simulink model "maglev"  (Simulink 3.00)
settings: Solver=ode45  StartTime=0.0  StopTime=10.0  RelTol=1e-3
values from neighbouring files (symbols this model uses):
  a = 0.2042    [mlevpar.m]
  b = 72.988    [mlevpar.m]
  g = 9.81    [mlevpar.m]
  mb = 0.0682    [mlevpar.m]
  yl = 0.02    [mlevpar.m]
settings Model: Creator=root

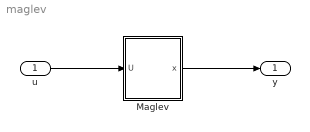
== system maglev ==
  u : Inport  Port=1  PortWidth=-1  SampleTime=-1  DataType=auto
      settings: SignalType=auto
  Maglev : Subsystem
  y : Outport  Port=1
  wires:
  Maglev/1(x) -> y/1
  u/1 -> Maglev/1(U)

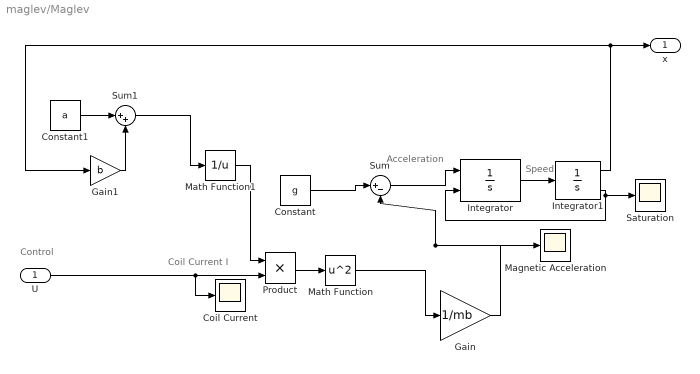
== system maglev/Maglev ==
  note: Control
  note: Speed
  note: Acceleration
  note: Coil Current I
  U : Inport  Port=1  PortWidth=-1  SampleTime=-1  DataType=auto
      settings: SignalType=auto
  Coil Current : Scope
      settings: TimeRange=auto  YMin=0  YMax=30  SaveToWorkspace=off  SaveName=ScopeData
  Constant : Constant  Value=g
  Constant1 : Constant  Value=a
  Gain : Gain  Gain=1/mb  SaturateOnIntegerOverflow=on
  Gain1 : Gain  Gain=b  SaturateOnIntegerOverflow=on
  Integrator : Integrator  ExternalReset=falling  InitialConditionSource=internal  InitialCondition=0  LimitOutput=off  UpperSaturationLimit=inf  LowerSaturationLimit=-inf  ShowSaturationPort=off  ShowStatePort=off  AbsoluteTolerance=auto
  Integrator1 : Integrator  ExternalReset=none  InitialConditionSource=internal  InitialCondition=yl  LimitOutput=on  UpperSaturationLimit=10  LowerSaturationLimit=0  ShowSaturationPort=on  ShowStatePort=off  AbsoluteTolerance=auto
  Magnetic Acceleration : Scope
      settings: TimeRange=auto  YMin=0  YMax=7  SaveToWorkspace=off  SaveName=ScopeData
  Math Function : Math  Operator=square  OutputSignalType=auto
  Math Function1 : Math  Operator=reciprocal  OutputSignalType=auto
  Product : Product  Inputs=2  SaturateOnIntegerOverflow=on
  Saturation : Scope
      settings: TimeRange=auto  YMin=0  YMax=7  SaveToWorkspace=off  SaveName=ScopeData  MaxRows=125000
  Sum : Sum  Inputs=|+-  SaturateOnIntegerOverflow=on
  Sum1 : Sum  Inputs=|++  SaturateOnIntegerOverflow=on
  x : Outport  Port=1
  wires:
  Gain/1 -> Magnetic Acceleration/1, Sum/2
  Product/1 -> Math Function/1
  Sum/1 -> Integrator/1
  Math Function1/1 -> Product/1
  Constant/1 -> Sum/1
  Sum1/1 -> Math Function1/1
  Gain1/1 -> Sum1/2
  Constant1/1 -> Sum1/1
  Integrator/1 -> Integrator1/1
  Math Function/1 -> Gain/1
  Integrator1/1 -> Gain1/1, x/1
  Integrator1/2 -> Integrator/2, Saturation/1
  U/1 -> Coil Current/1, Product/2
